simulink model "PMSM_Simscape_Model"  (R2020b)
settings: configuration reference "SLRT" (kept outside this file)
PreLoadFcn:
  | % Load modeSchedulerEnum if required
  | if ~exist('modeSchedulerEnum','class')
  |   load_system('ModeLogicModule');
  | end
undefined symbols (not defined in the file): adc, boardResistance, discInertia, encoder, inverter, pmsm, pmsmInertia, pwm
libraries: fl_lib x18, nesl_utility x10, ee_lib x3, eeTransforms x1
settings Model: DataDictionary=SGKitPlantData.sldd  EnableAccessToBaseWorkspace=off  OrderedModelArguments=off  Creator=promero  LastModifiedBy=manuel.fedou
settings ConfigSetRef: SourceName=SLRT

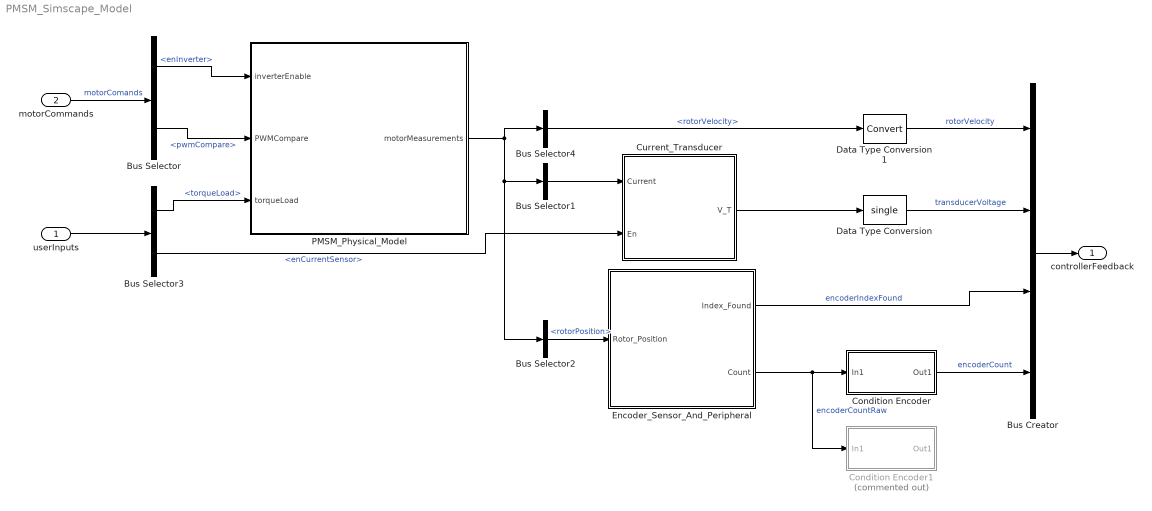
== system PMSM_Simscape_Model ==
  userInputs : Inport  OutDataTypeStr=Bus: userInputs  PortDimensions=1
  motorCommands : Inport  Port=2  OutDataTypeStr=Bus: motorCommands
  Bus Creator : BusCreator  Inputs=4  OutDataTypeStr=Bus: controllerFeedback
      settings: InheritFromInputs=off
  Bus Selector : BusSelector  OutputSignals=enInverter,pwmCompare
  Bus Selector1 : BusSelector  OutputSignals=phaseCurrentA,phaseCurrentB  OutputAsBus=on
  Bus Selector2 : BusSelector  OutputSignals=rotorPosition
  Bus Selector3 : BusSelector  OutputSignals=torqueLoad,enCurrentSensor
  Bus Selector4 : BusSelector  OutputSignals=rotorVelocity
  Condition Encoder : Subsystem  mask(Speedgoat Encoder Counter){cntsPerRevolution=encoder.CountPerRevolution, positiveDirection=encoder.ALeadsB}
      mask prompts: cntsPerRevolution "Counts per revolution"; positiveDirection "A leads B?"
      mask help: Configures the direction and positive range of the counter value returned by the Speedgoat IO313 QAD Read block.
      mask init:
      | if positiveDirection == 1
      |     strPositiveDirection = 'A Leads B';
      | else
      |     strPositiveDirection = 'B Leads A';
      | end
      mask Display: fprintf(['Encoder\nPositive Direction:\n' strPositiveDirection]);
  Condition Encoder1 : Subsystem  Commented=on  mask(Speedgoat Encoder Counter){cntsPerRevolution=encoder.CountPerRevolution, positiveDirection=encoder.ALeadsB}
      mask prompts: cntsPerRevolution "Counts per revolution"; positiveDirection "A leads B?"
      mask help: Configures the direction and positive range of the counter value returned by the Speedgoat IO313 QAD Read block.
      mask init:
      | if positiveDirection == 1
      |     strPositiveDirection = 'A Leads B';
      | else
      |     strPositiveDirection = 'B Leads A';
      | end
      mask Display: fprintf(['Encoder\nPositive Direction:\n' strPositiveDirection]);
  Current_Transducer : Subsystem
      mask Display: image('currentTransducerMask.png');
  Data Type Conversion : DataTypeConversion  OutDataTypeStr=single
  Data Type Conversion1 : DataTypeConversion
  Encoder_Sensor_And_Peripheral : Subsystem
      mask Display:
      | image('encoderSensorAndPeripheralMask.png')
      | port_label('input',1,'P')
      | port_label('output',1,sprintf('Index\nFound'))
      | port_label('output',2,'Count')
  PMSM_Physical_Model : Subsystem
      mask Display: image('focVelocityMotorAndLoadMask.png');
  controllerFeedback : Outport  OutDataTypeStr=Bus: controllerFeedback  VectorParamsAs1DForOutWhenUnconnected=off
  wires:
  Bus Selector3/1 -> PMSM_Physical_Model/3(torqueLoad)  "<torqueLoad>"
  Bus Selector2/1 -> Encoder_Sensor_And_Peripheral/1(Rotor_Position)  "<rotorPosition>"
  Bus Selector/2 -> PMSM_Physical_Model/2(PWMCompare)  "<pwmCompare>"
  motorCommands/1 -> Bus Selector/1  "motorComands"
  Encoder_Sensor_And_Peripheral/2(Count) -> Condition Encoder1/1(In1), Condition Encoder/1(In1)  "encoderCountRaw"
  Encoder_Sensor_And_Peripheral/1(Index_Found) -> Bus Creator/3  "encoderIndexFound"
  Bus Selector3/2 -> Current_Transducer/2(En)  "<enCurrentSensor>"
  Condition Encoder/1(Out1) -> Bus Creator/4  "encoderCount"
  Bus Selector1/1 -> Current_Transducer/1(Current)
  Bus Selector/1 -> PMSM_Physical_Model/1(inverterEnable)  "<enInverter>"
  userInputs/1 -> Bus Selector3/1
  Bus Creator/1 -> controllerFeedback/1
  PMSM_Physical_Model/1(motorMeasurements) -> Bus Selector4/1, Bus Selector2/1, Bus Selector1/1
  Current_Transducer/1(V_T) -> Data Type Conversion/1
  Data Type Conversion/1 -> Bus Creator/2  "transducerVoltage"
  Bus Selector4/1 -> Data Type Conversion1/1  "<rotorVelocity>"
  Data Type Conversion1/1 -> Bus Creator/1  "rotorVelocity"

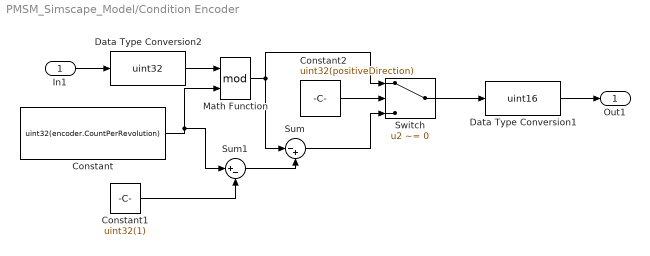
== system PMSM_Simscape_Model/Condition Encoder ==
  In1 : Inport
  Constant : Constant  Value=uint32(encoder.CountPerRevolution)  OutDataTypeStr=uint32
  Constant1 : Constant  Value=uint32(1)
  Constant2 : Constant  Value=uint32(positiveDirection)
  Data Type Conversion1 : DataTypeConversion  OutDataTypeStr=uint16
  Data Type Conversion2 : DataTypeConversion  OutDataTypeStr=uint32
  Math Function : Math  Operator=mod  SignedPower=on  SaturateOnIntegerOverflow=on
  Sum : Sum  Inputs=|-+
  Sum1 : Sum  Inputs=|+-
  Switch : Switch  Criteria=u2 ~= 0
  Out1 : Outport  VectorParamsAs1DForOutWhenUnconnected=off
  wires:
  Math Function/1 -> Sum/1, Switch/1
  Constant/1 -> Math Function/2, Sum1/1
  In1/1 -> Data Type Conversion2/1
  Data Type Conversion1/1 -> Out1/1
  Constant1/1 -> Sum1/2
  Sum1/1 -> Sum/2
  Constant2/1 -> Switch/2
  Sum/1 -> Switch/3
  Switch/1 -> Data Type Conversion1/1
  Data Type Conversion2/1 -> Math Function/1

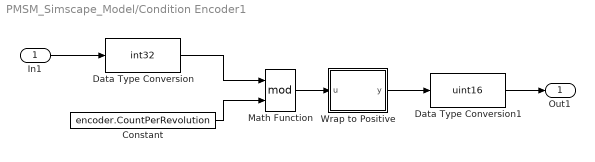
== system PMSM_Simscape_Model/Condition Encoder1 ==
  In1 : Inport
  Constant : Constant  Value=encoder.CountPerRevolution  OutDataTypeStr=int32
  Data Type Conversion : DataTypeConversion  OutDataTypeStr=int32
  Data Type Conversion1 : DataTypeConversion  OutDataTypeStr=uint16
  Math Function : Math  Operator=mod  SignedPower=on  SaturateOnIntegerOverflow=on
  Wrap to Positive : MATLAB Function  TreatAsAtomicUnit=on
  Out1 : Outport  VectorParamsAs1DForOutWhenUnconnected=off
  wires:
  Math Function/1 -> Wrap to Positive/1(u)
  Constant/1 -> Math Function/2
  In1/1 -> Data Type Conversion/1
  Wrap to Positive/1(y) -> Data Type Conversion1/1
  Data Type Conversion/1 -> Math Function/1
  Data Type Conversion1/1 -> Out1/1

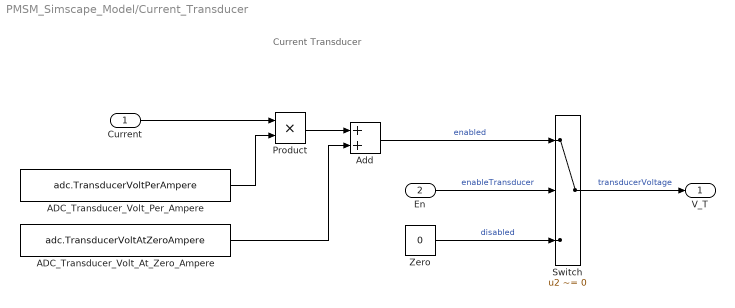
== system PMSM_Simscape_Model/Current_Transducer ==
  note: Current Transducer
  Current : Inport
  En : Inport  Port=2
  ADC_Transducer_Volt_At_Zero_Ampere : Constant  Value=adc.TransducerVoltAtZeroAmpere
  ADC_Transducer_Volt_Per_Ampere : Constant  Value=adc.TransducerVoltPerAmpere
  Add : Sum
  Product : Product  RndMeth=Zero
  Switch : Switch  Criteria=u2 ~= 0
  Zero : Constant  Value=0
  V_T : Outport  VectorParamsAs1DForOutWhenUnconnected=off
  wires:
  Current/1 -> Product/1
  ADC_Transducer_Volt_At_Zero_Ampere/1 -> Add/2
  Product/1 -> Add/1
  ADC_Transducer_Volt_Per_Ampere/1 -> Product/2
  Zero/1 -> Switch/3  "disabled"
  Switch/1 -> V_T/1  "transducerVoltage"
  Add/1 -> Switch/1  "enabled"
  En/1 -> Switch/2  "enableTransducer"

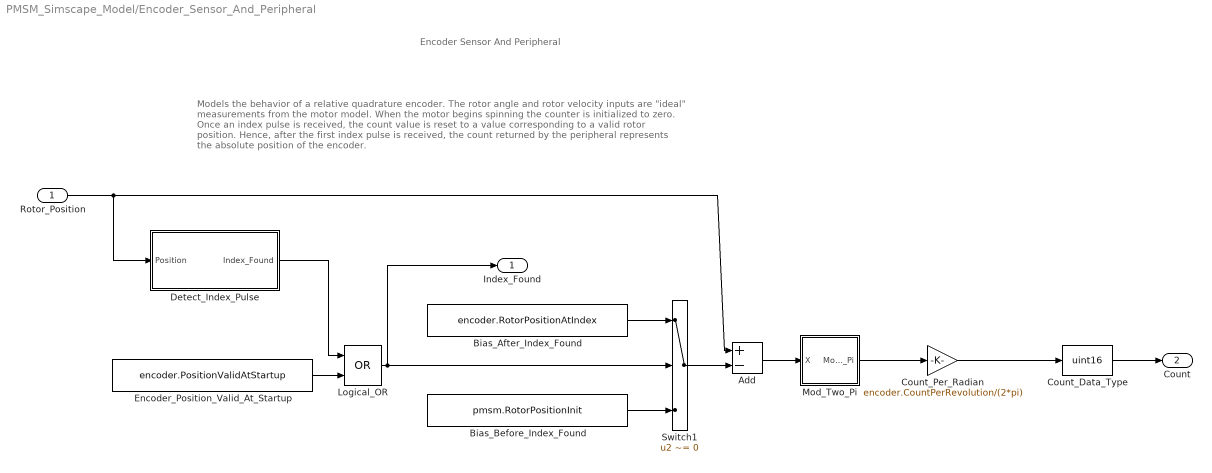
== system PMSM_Simscape_Model/Encoder_Sensor_And_Peripheral ==
  note: Models the behavior of a relative quadrature encoder. The rotor angle and rotor velocity inputs are "ideal" measurements from the motor model.
      | When the motor begins spinning the counter is initialized to zero.
      | Once an index pulse is received, the count value is reset to a value corresponding to a valid rotor position.
      | Hence, after the first index pulse is received, the count returned by the peripheral represents the absolute position of the encoder.
  note: Encoder Sensor And Peripheral
  Rotor_Position : Inport
  Add : Sum  Inputs=+-
  Bias_After_Index_Found : Constant  Value=encoder.RotorPositionAtIndex
  Bias_Before_Index_Found : Constant  Value=pmsm.RotorPositionInit
  Count_Data_Type : DataTypeConversion  OutDataTypeStr=uint16
  Count_Per_Radian : Gain  Gain=encoder.CountPerRevolution/(2*pi)
      settings: AttributesFormatString=|
      | ------------------------------------------
      | Gain = %<Gain>
  Detect_Index_Pulse : Subsystem
  Encoder_Position_Valid_At_Startup : Constant  Value=encoder.PositionValidAtStartup
  Logical_OR : Logic  Operator=OR  IconShape=distinctive  AllPortsSameDT=off  OutDataTypeStr=boolean
  Mod_Two_Pi : Subsystem
      mask Display:
      | text(0.5, 0.5,'Mod 2\pi',...
      |   'HorizontalAlignment', 'Center',...
      |   'VerticalAlignment', 'Middle',...
      |   'texmode', 'on')
  Switch1 : Switch  Criteria=u2 ~= 0
  Index_Found : Outport  VectorParamsAs1DForOutWhenUnconnected=off
  Count : Outport  Port=2  VectorParamsAs1DForOutWhenUnconnected=off
  wires:
  Bias_Before_Index_Found/1 -> Switch1/3
  Bias_After_Index_Found/1 -> Switch1/1
  Logical_OR/1 -> Index_Found/1, Switch1/2
  Encoder_Position_Valid_At_Startup/1 -> Logical_OR/2
  Detect_Index_Pulse/1(Index_Found) -> Logical_OR/1
  Rotor_Position/1 -> Add/1, Detect_Index_Pulse/1(Position)
  Mod_Two_Pi/1(Mod_X_Two_Pi) -> Count_Per_Radian/1
  Count_Data_Type/1 -> Count/1
  Switch1/1 -> Add/2
  Add/1 -> Mod_Two_Pi/1(X)
  Count_Per_Radian/1 -> Count_Data_Type/1

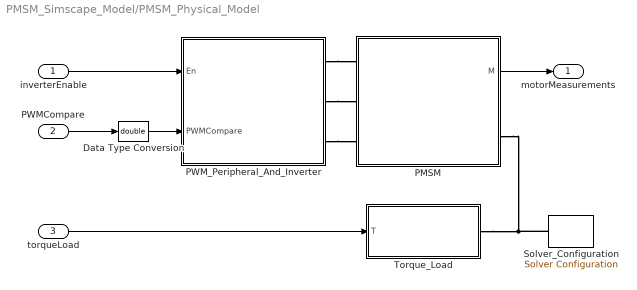
== system PMSM_Simscape_Model/PMSM_Physical_Model ==
  inverterEnable : Inport
  PWMCompare : Inport  Port=2
  torqueLoad : Inport  Port=3
  Data Type Conversion : DataTypeConversion  OutDataTypeStr=double
  PMSM : Subsystem
      mask Display:
      | image('pmsmMask.png')
      | text(0.03, 0.80, 'A', 'HorizontalAlignment', 'Left')
      | text(0.03, 0.50, 'B', 'HorizontalAlignment', 'Left')
      | text(0.03, 0.20, 'C', 'HorizontalAlignment', 'Left')
      | text(0.98, 0.75, 'M', 'HorizontalAlignment', 'Right')
      | text(0.98, 0.25, 'R', 'HorizontalAlignment', 'Right')
  PWM_Peripheral_And_Inverter : Subsystem  VariantControl=variantPwm == enumPwm.behavior
      mask Display: image('pwmPeripheralAndInverterMask.png');
  Solver_Configuration : nesl_utility/Solver Configuration  PhysicalDomain=network_engine_domain  SubClassName=solver  LeftPortType=input  RightPortType=generic  Tones=[]  Harmonics=[]  SimulateNoise=off  Profile=off  UseLocalSampling=off  EnableSwitchedLinearOptims=on  FrequencyDomain=off  UseCCode=off  RelTol=0.001  AbsTol=1e-06  MinStep=1e-09  ToWorkspace=off  RevertToSquareIcSolve=off  NumHomotopyIterations=100  PhasorMode=off  PhasorModeNumHarmonics=1  DoDC=off  ResidualTolerance=1e-9  UseLocalSolver=on  LocalSolverChoice=NE_BACKWARD_EULER_ADVANCER  LocalSolverSampleTime=sampleTime.CurrentControl  DoFixedCost=on  MaxNonlinIter=1  MaxModeIter=2  ComputeImpulses=off  ImpulseIterations=2  LinearAlgebra=auto  EquationFormulation=NE_TIME_EF  DelaysMemoryBudget=1024  AutomaticFiltering=off  FilteringTimeConstant=0.001  PartitionStorageMethod=EXHAUSTIVE  PartitionMemoryBudget=1024  PartitionMethod=FAST
  Torque_Load : Subsystem  VariantControl=loadType == motorLoad.disc
      mask Display:
      | image('torqueLoadMask.png')
      | text(0.03, 0.5, 'T', 'HorizontalAlignment', 'Left')
      | text(0.98, 0.5, 'R', 'HorizontalAlignment', 'Right')
  motorMeasurements : Outport  VectorParamsAs1DForOutWhenUnconnected=off
  wires:
  PWMCompare/1 -> Data Type Conversion/1
  torqueLoad/1 -> Torque_Load/1(T)
  PMSM/1(M) -> motorMeasurements/1
  inverterEnable/1 -> PWM_Peripheral_And_Inverter/1(En)
  Data Type Conversion/1 -> PWM_Peripheral_And_Inverter/2(PWMCompare)
  connections:
  Solver_Configuration/RConn1 -- PMSM/RConn1 -- Torque_Load/RConn1
  PWM_Peripheral_And_Inverter/RConn3 -- PMSM/LConn3
  PWM_Peripheral_And_Inverter/RConn2 -- PMSM/LConn2
  PWM_Peripheral_And_Inverter/RConn1 -- PMSM/LConn1

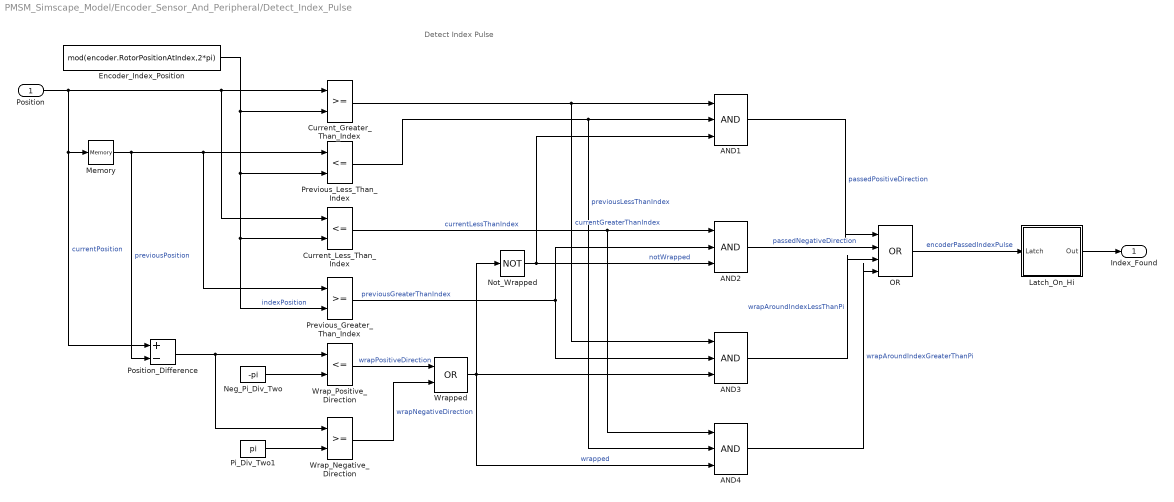
== system PMSM_Simscape_Model/Encoder_Sensor_And_Peripheral/Detect_Index_Pulse ==
  note: Detect Index Pulse
  Position : Inport
  AND{1..4} (4 alike) : Logic  Inputs=3  IconShape=distinctive  AllPortsSameDT=off  OutDataTypeStr=boolean
  Current_Greater_Than_Index : RelationalOperator  OutDataTypeStr=boolean  RndMeth=Nearest
  Current_Less_Than_Index : RelationalOperator  Operator=<=  OutDataTypeStr=boolean  RndMeth=Nearest
  Encoder_Index_Position : Constant  Value=mod(encoder.RotorPositionAtIndex,2*pi)
  Latch_On_Hi : Subsystem
  Memory : Memory  InheritSampleTime=on
  Neg_Pi_Div_Two : Constant  Value=-pi
  Not_Wrapped : Logic  Operator=NOT  IconShape=distinctive  AllPortsSameDT=off  OutDataTypeStr=boolean
  OR : Logic  Operator=OR  Inputs=4  IconShape=distinctive  AllPortsSameDT=off  OutDataTypeStr=boolean
  Pi_Div_Two1 : Constant  Value=pi
  Position_Difference : Sum  Inputs=+-
  Previous_Greater_Than_Index : RelationalOperator  OutDataTypeStr=boolean  RndMeth=Nearest
  Previous_Less_Than_Index : RelationalOperator  Operator=<=  OutDataTypeStr=boolean  RndMeth=Nearest
  Wrap_Negative_Direction : RelationalOperator  OutDataTypeStr=boolean  RndMeth=Nearest
  Wrap_Positive_Direction : RelationalOperator  Operator=<=  OutDataTypeStr=boolean  RndMeth=Nearest
  Wrapped : Logic  Operator=OR  IconShape=distinctive  AllPortsSameDT=off  OutDataTypeStr=boolean
  Index_Found : Outport  VectorParamsAs1DForOutWhenUnconnected=off
  wires:
  AND2/1 -> OR/2  "passedNegativeDirection"
  AND1/1 -> OR/1  "passedPositiveDirection"
  Current_Less_Than_Index/1 -> AND2/1, AND4/1  "currentLessThanIndex"
  Previous_Greater_Than_Index/1 -> AND2/2, AND3/2  "previousGreaterThanIndex"
  OR/1 -> Latch_On_Hi/1(Latch)  "encoderPassedIndexPulse"
  Encoder_Index_Position/1 -> Previous_Less_Than_Index/2, Previous_Greater_Than_Index/2, Current_Less_Than_Index/2, Current_Greater_Than_Index/2  "indexPosition"
  Previous_Less_Than_Index/1 -> AND1/2, AND4/2  "previousLessThanIndex"
  Current_Greater_Than_Index/1 -> AND3/1, AND1/1  "currentGreaterThanIndex"
  Memory/1 -> Position_Difference/2, Previous_Greater_Than_Index/1, Previous_Less_Than_Index/1  "previousPosition"
  Position/1 -> Memory/1, Position_Difference/1, Current_Less_Than_Index/1, Current_Greater_Than_Index/1  "currentPosition"
  Position_Difference/1 -> Wrap_Negative_Direction/1, Wrap_Positive_Direction/1
  Wrap_Positive_Direction/1 -> Wrapped/1  "wrapPositiveDirection"
  Neg_Pi_Div_Two/1 -> Wrap_Positive_Direction/2
  Wrap_Negative_Direction/1 -> Wrapped/2  "wrapNegativeDirection"
  Pi_Div_Two1/1 -> Wrap_Negative_Direction/2
  AND3/1 -> OR/3  "wrapAroundIndexLessThanPi"
  Latch_On_Hi/1(Out) -> Index_Found/1
  Not_Wrapped/1 -> AND1/3, AND2/3  "notWrapped"
  Wrapped/1 -> AND4/3, AND3/3, Not_Wrapped/1  "wrapped"
  AND4/1 -> OR/4  "wrapAroundIndexGreaterThanPi"

== system PMSM_Simscape_Model/Encoder_Sensor_And_Peripheral/Mod_Two_Pi ==
  note: Mod Two Pi
  X : Inport
  Mod : Math  Operator=mod  SignedPower=on  SaturateOnIntegerOverflow=on
  Two_Pi : Constant  Value=2*pi  OutDataTypeStr=Inherit: Inherit via back propagation
  Mod_X_Two_Pi : Outport  VectorParamsAs1DForOutWhenUnconnected=off
  wires:
  X/1 -> Mod/1
  Two_Pi/1 -> Mod/2
  Mod/1 -> Mod_X_Two_Pi/1

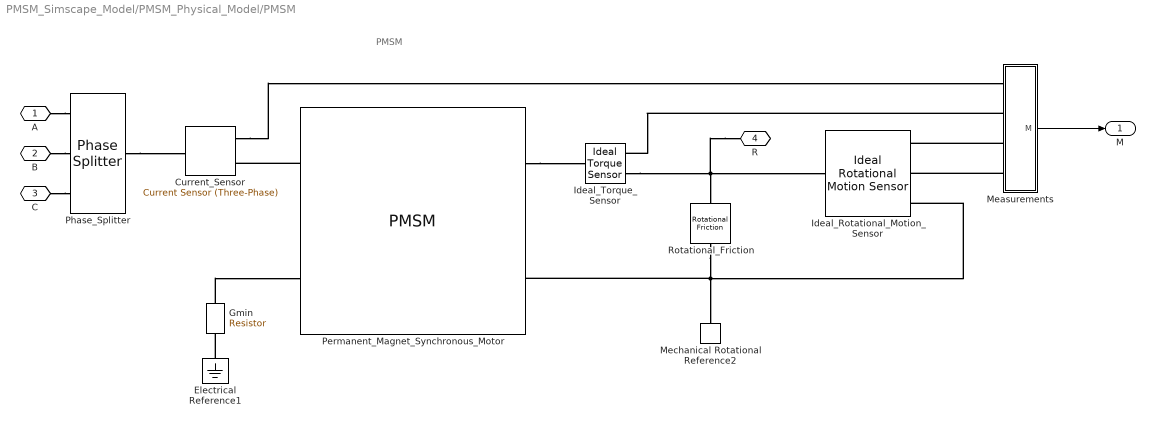
== system PMSM_Simscape_Model/PMSM_Physical_Model/PMSM ==
  note: PMSM
  Current_Sensor : ee_lib/Sensors & Transducers/Current Sensor (Three-Phase)
  Electrical Reference1 : fl_lib/Electrical/Electrical Elements/Electrical Reference
  Gmin : fl_lib/Electrical/Electrical Elements/Resistor  R=1e9 Ohm  i_specify=off  i_priority=None  i=0 A  i_nominal_specify=off  i_nominal_unit=A  i_nominal_value=1  v_specify=off  v_priority=None  v=0 V  v_nominal_specify=off  v_nominal_unit=V  v_nominal_value=1
  Ideal_Rotational_Motion_Sensor : fl_lib/Mechanical/Mechanical Sensors/Ideal Rotational Motion Sensor  wrap_angle=simscape.enum.onoff.off  offset=pmsm.RotorPositionInit rad
  Ideal_Torque_Sensor : fl_lib/Mechanical/Mechanical Sensors/Ideal Torque Sensor
  Measurements : Subsystem
  Mechanical Rotational Reference2 : fl_lib/Mechanical/Rotational Elements/Mechanical Rotational Reference
  Permanent_Magnet_Synchronous_Motor : ee_lib/Electromechanical/Permanent Magnet/PMSM  winding_type=ee.enum.statorconnection.wye  machine_param=ee.enum.pmsm.parameterization.constant  nPolePairs=pmsm.PolePairs  pmflux_param=ee.enum.pmflux.fluxlinkage  pm_flux_linkage=pmsm.FluxLinkage Wb  torque_constant=pmsm.TorqueConstant N*m/A  back_emf_constant=0.18 V/(rad/s)  stator_param=ee.enum.statorparam.LdLqL0  Ld=pmsm.InductanceLd H  Lq=pmsm.InductanceLq H  idVec=[-200, 0, 200] A  iqVec=[-200, 0, 200] A  LdMatrix=0.0002 * ones(3, 3) H  LqMatrix=0.0002 * ones(3, 3) H  PmMatrix=0.1 * ones(3, 3) Wb  ktMatrix=0.18 * ones(3, 3) N*m/A  keMatrix=0.18 * ones(3, 3) V/(rad/s)  L0=pmsm.InductanceL0 H  Ls=0.0002 H  Lm=0 H  Ms=0 H  Rs=pmsm.StatorPhaseResistance Ohm  zero_sequence=ee.enum.park.zerosequence.exclude  J=pmsmInertia+discInertia kg*m^2  lam=0 N*m/(rad/s)  axes_param=ee.enum.rotorangle.daxis  i_d_specify=off  i_d_priority=None  i_d=0 A  i_d_nominal_specify=off  i_d_nominal_unit=A  i_d_nominal_value=1  i_q_specify=off  i_q_priority=None  i_q=0 A  i_q_nominal_specify=off  i_q_nominal_unit=A  i_q_nominal_value=1  torque_specify=off  torque_priority=None  torque=0 N*m  torque_nominal_specify=off  torque_nominal_unit=N*m  torque_nominal_value=1  angular_velocity_specify=on  angular_velocity_priority=High  angular_velocity=pmsm.RotorVelocityInit rad/s  angular_velocity_nominal_specify=off  angular_velocity_nominal_unit=rpm  angular_velocity_nominal_value=1  angular_position_specify=on  angular_position_priority=High  angular_position=pmsm.RotorPositionInit rad  angular_position_nominal_specify=off  angular_position_nominal_unit=deg  angular_position_nominal_value=1  loss_param=ee.enum.ironloss.none  losses_oc=[0, 0, 0] W  losses_sc=[0, 0, 0] W  f_losses=60 Hz  Isc_losses=95 A  Tmeas=298.15 K  alpha=3.93e-3 1/K  alpha_flux=-0.001 1/K  stator_thermal_mass=100 J/K  rotor_thermal_mass=200 J/K  Rm_percent_rotor=90  Rd_percent_rotor=30  temperatureA_specify=off  temperatureA_priority=High  temperatureA=25 degC  temperatureA_nominal_specify=off  temperatureA_nominal_unit=degC  temperatureA_nominal_value=1  temperatureB_specify=off  temperatureB_priority=High  temperatureB=25 degC  temperatureB_nominal_specify=off  temperatureB_nominal_unit=degC  temperatureB_nominal_value=1  temperatureC_specify=off  temperatureC_priority=High  temperatureC=25 degC  temperatureC_nominal_specify=off  temperatureC_nominal_unit=degC  temperatureC_nominal_value=1  temperatureR_specify=off  temperatureR_priority=High  temperatureR=25 degC  temperatureR_nominal_specify=off  temperatureR_nominal_unit=degC  temperatureR_nominal_value=1
      settings: InternalSimscapePortConfiguration="{\"Bottom\":[],\"Left\":[{\"id\":\"N\",\"label\":\"~\",\"type\":\"foundation.electrical.three_phase\"},{\"id\":\"n\",\"label\":\"n\",\"type\":\"foundation.electrical.electrical\"}],\"Right\":[{\"id\":\"R\",\"label\":\"R\",\"type\":\"foundation.mechanical.rotational.rotational\"},{\"id\":\"C\",\"label\":\"C\",\"type\":\"foundation.mechanical.rotational.rotational\"}],\"Top\":[]}"
  Phase_Splitter : ee_lib/Connectors & References/Phase Splitter
      settings: SourceProductBaseCode=PS
  Rotational_Friction : fl_lib/Mechanical/Rotational Elements/Rotational Friction  brkwy_trq=pmsmBreakawayFrictionTorque N*m  brkwy_vel=pmsmBreakawayFrictionVelocity rad/s  Col_trq=pmsmCoulombFrictionTorque N*m  visc_coef=pmsmViscousFrictionCoefficient N*m/(rad/s)  w_specify=off  w_priority=None  w=0 rad/s  w_nominal_specify=off  w_nominal_unit=rad/s  w_nominal_value=1  t_specify=off  t_priority=None  t=0 N*m  t_nominal_specify=off  t_nominal_unit=N*m  t_nominal_value=1
  A : PMIOPort  Side=Left
  B : PMIOPort  Port=2  Side=Left
  C : PMIOPort  Port=3  Side=Left
  R : PMIOPort  Port=4  Side=Right
  M : Outport  VectorParamsAs1DForOutWhenUnconnected=off
  wires:
  Measurements/1(M) -> M/1
  connections:
  Measurements/LConn4 -- Ideal_Rotational_Motion_Sensor/RConn2
  Measurements/LConn3 -- Ideal_Rotational_Motion_Sensor/RConn3
  Measurements/LConn2 -- Ideal_Torque_Sensor/RConn2
  Permanent_Magnet_Synchronous_Motor/LConn1 -- Current_Sensor/RConn2
  C/RConn1 -- Phase_Splitter/RConn3
  B/RConn1 -- Phase_Splitter/RConn2
  A/RConn1 -- Phase_Splitter/RConn1
  Gmin/RConn1 -- Permanent_Magnet_Synchronous_Motor/LConn2
  Permanent_Magnet_Synchronous_Motor/RConn2 -- Rotational_Friction/RConn1 -- Ideal_Rotational_Motion_Sensor/RConn1 -- Mechanical Rotational Reference2/LConn1
  Phase_Splitter/LConn1 -- Current_Sensor/LConn1
  Current_Sensor/RConn1 -- Measurements/LConn1
  Electrical Reference1/LConn1 -- Gmin/LConn1
  Permanent_Magnet_Synchronous_Motor/RConn1 -- Ideal_Torque_Sensor/LConn1
  R/RConn1 -- Ideal_Rotational_Motion_Sensor/LConn1 -- Ideal_Torque_Sensor/RConn1 -- Rotational_Friction/LConn1

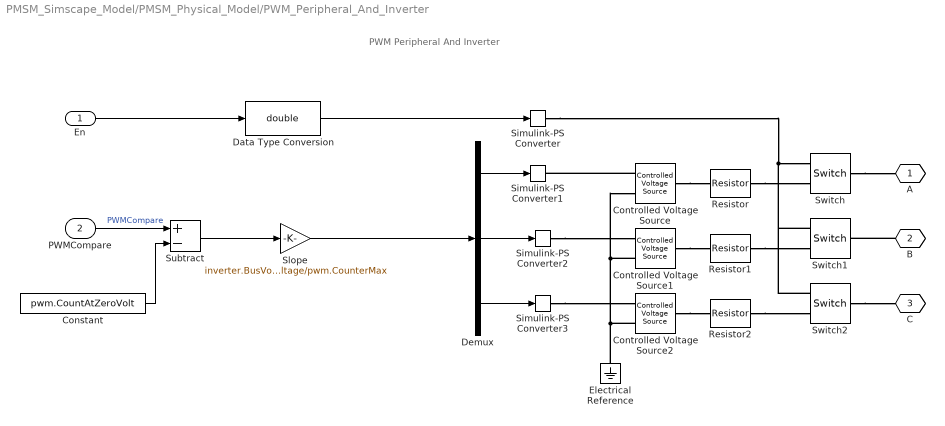
== system PMSM_Simscape_Model/PMSM_Physical_Model/PWM_Peripheral_And_Inverter ==
  note: PWM Peripheral And Inverter
  En : Inport
  PWMCompare : Inport  Port=2
  Constant : Constant  Value=pwm.CountAtZeroVolt  SampleTime=-1
  Controlled Voltage Source : fl_lib/Electrical/Electrical Sources/Controlled Voltage Source
  Controlled Voltage Source1 : fl_lib/Electrical/Electrical Sources/Controlled Voltage Source
  Controlled Voltage Source2 : fl_lib/Electrical/Electrical Sources/Controlled Voltage Source
  Data Type Conversion : DataTypeConversion  OutDataTypeStr=double
  Demux : Demux  Outputs=3
  Electrical Reference : fl_lib/Electrical/Electrical Elements/Electrical Reference
  Resistor : fl_lib/Electrical/Electrical Elements/Resistor  R=boardResistance Ohm  i_specify=off  i_priority=None  i=0 A  i_nominal_specify=off  i_nominal_unit=A  i_nominal_value=1  v_specify=off  v_priority=None  v=0 V  v_nominal_specify=off  v_nominal_unit=V  v_nominal_value=1
  Resistor1 : fl_lib/Electrical/Electrical Elements/Resistor  R=boardResistance Ohm  i_specify=off  i_priority=None  i=0 A  i_nominal_specify=off  i_nominal_unit=A  i_nominal_value=1  v_specify=off  v_priority=None  v=0 V  v_nominal_specify=off  v_nominal_unit=V  v_nominal_value=1
  Resistor2 : fl_lib/Electrical/Electrical Elements/Resistor  R=boardResistance Ohm  i_specify=off  i_priority=None  i=0 A  i_nominal_specify=off  i_nominal_unit=A  i_nominal_value=1  v_specify=off  v_priority=None  v=0 V  v_nominal_specify=off  v_nominal_unit=V  v_nominal_value=1
  Simulink-PS Converter : nesl_utility/Simulink-PS Converter  PhysicalDomain=network_engine_domain  SubClassName=ps_input  LeftPortType=input  RightPortType=output  PseudoPeriodic=off  Frequencies=[]  NoiseDistribution=none  NoiseParameters=[]  Unit=1  AffineConversion=off  FilteringAndDerivatives=provide  SimscapeFilterOrder=1  InputFilterTimeConstant=0.001  UdotUserProvided=0
  Simulink-PS Converter1 : nesl_utility/Simulink-PS Converter  PhysicalDomain=network_engine_domain  SubClassName=ps_input  LeftPortType=input  RightPortType=output  PseudoPeriodic=off  Frequencies=[]  NoiseDistribution=none  NoiseParameters=[]  Unit=V  AffineConversion=off  FilteringAndDerivatives=provide  SimscapeFilterOrder=1  InputFilterTimeConstant=0.001  UdotUserProvided=0
  Simulink-PS Converter2 : nesl_utility/Simulink-PS Converter  PhysicalDomain=network_engine_domain  SubClassName=ps_input  LeftPortType=input  RightPortType=output  PseudoPeriodic=off  Frequencies=[]  NoiseDistribution=none  NoiseParameters=[]  Unit=V  AffineConversion=off  FilteringAndDerivatives=provide  SimscapeFilterOrder=1  InputFilterTimeConstant=0.001  UdotUserProvided=0
  Simulink-PS Converter3 : nesl_utility/Simulink-PS Converter  PhysicalDomain=network_engine_domain  SubClassName=ps_input  LeftPortType=input  RightPortType=output  PseudoPeriodic=off  Frequencies=[]  NoiseDistribution=none  NoiseParameters=[]  Unit=V  AffineConversion=off  FilteringAndDerivatives=provide  SimscapeFilterOrder=1  InputFilterTimeConstant=0.001  UdotUserProvided=0
  Slope : Gain  Gain=inverter.BusVoltage/pwm.CounterMax
      settings: AttributesFormatString=|
      | ----------------------------------------
      | Gain = %<Gain>
  Subtract : Sum  Inputs=+-
  Switch : fl_lib/Electrical/Electrical Elements/Switch  R_closed=0.01 Ohm  G_open=1e-8 1/Ohm  Threshold=0.5  i_specify=off  i_priority=None  i=0 A  i_nominal_specify=off  i_nominal_unit=A  i_nominal_value=1  v_specify=off  v_priority=None  v=0 V  v_nominal_specify=off  v_nominal_unit=V  v_nominal_value=1
  Switch1 : fl_lib/Electrical/Electrical Elements/Switch  R_closed=0.01 Ohm  G_open=1e-8 1/Ohm  Threshold=0.5  i_specify=off  i_priority=None  i=0 A  i_nominal_specify=off  i_nominal_unit=A  i_nominal_value=1  v_specify=off  v_priority=None  v=0 V  v_nominal_specify=off  v_nominal_unit=V  v_nominal_value=1
  Switch2 : fl_lib/Electrical/Electrical Elements/Switch  R_closed=0.01 Ohm  G_open=1e-8 1/Ohm  Threshold=0.5  i_specify=off  i_priority=None  i=0 A  i_nominal_specify=off  i_nominal_unit=A  i_nominal_value=1  v_specify=off  v_priority=None  v=0 V  v_nominal_specify=off  v_nominal_unit=V  v_nominal_value=1
  A : PMIOPort  Tag=PMCPort  Side=Right
  B : PMIOPort  Tag=PMCPort  Port=2  Side=Right
  C : PMIOPort  Tag=PMCPort  Port=3  Side=Right
  wires:
  En/1 -> Data Type Conversion/1
  Slope/1 -> Demux/1
  PWMCompare/1 -> Subtract/1  "PWMCompare"
  Demux/1 -> Simulink-PS Converter1/1
  Demux/2 -> Simulink-PS Converter2/1
  Demux/3 -> Simulink-PS Converter3/1
  Data Type Conversion/1 -> Simulink-PS Converter/1
  Subtract/1 -> Slope/1
  Constant/1 -> Subtract/2
  connections:
  Controlled Voltage Source2/LConn1 -- Resistor2/LConn1
  Resistor1/RConn1 -- Switch1/RConn2
  Resistor/RConn1 -- Switch/RConn2
  Electrical Reference/LConn1 -- Controlled Voltage Source1/RConn2 -- Controlled Voltage Source/RConn2 -- Controlled Voltage Source2/RConn2
  Switch/LConn1 -- A/RConn1
  B/RConn1 -- Switch1/LConn1
  Simulink-PS Converter/RConn1 -- Switch2/RConn1 -- Switch1/RConn1 -- Switch/RConn1
  Switch2/LConn1 -- C/RConn1
  Controlled Voltage Source/RConn1 -- Simulink-PS Converter1/RConn1
  Simulink-PS Converter2/RConn1 -- Controlled Voltage Source1/RConn1
  Simulink-PS Converter3/RConn1 -- Controlled Voltage Source2/RConn1
  Controlled Voltage Source/LConn1 -- Resistor/LConn1
  Controlled Voltage Source1/LConn1 -- Resistor1/LConn1
  Resistor2/RConn1 -- Switch2/RConn2

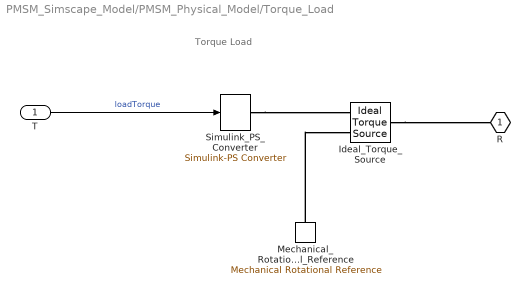
== system PMSM_Simscape_Model/PMSM_Physical_Model/Torque_Load ==
  note: Torque Load
  T : Inport
  Ideal_Torque_Source : fl_lib/Mechanical/Mechanical Sources/Ideal Torque Source
  Mechanical_Rotational_Reference : fl_lib/Mechanical/Rotational Elements/Mechanical Rotational Reference
  Simulink_PS_Converter : nesl_utility/Simulink-PS Converter  PhysicalDomain=network_engine_domain  SubClassName=ps_input  LeftPortType=input  RightPortType=output  PseudoPeriodic=off  Frequencies=[]  NoiseDistribution=none  NoiseParameters=[]  Unit=N*m  AffineConversion=off  FilteringAndDerivatives=zero  SimscapeFilterOrder=1  InputFilterTimeConstant=.001  UdotUserProvided=0
  R : PMIOPort  Side=Right
  wires:
  T/1 -> Simulink_PS_Converter/1  "loadTorque"
  connections:
  Ideal_Torque_Source/LConn1 -- R/RConn1
  Simulink_PS_Converter/RConn1 -- Ideal_Torque_Source/RConn1
  Mechanical_Rotational_Reference/LConn1 -- Ideal_Torque_Source/RConn2

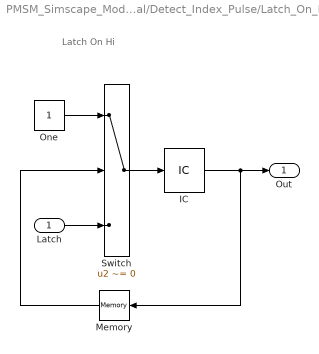
== system PMSM_Simscape_Model/Encoder_Sensor_And_Peripheral/Detect_Index_Pulse/Latch_On_Hi ==
  note: Latch On Hi
  Latch : Inport
  IC : InitialCondition  Value=0
  Memory : Memory  InheritSampleTime=on
  One : Constant  OutDataTypeStr=boolean
  Switch : Switch  Criteria=u2 ~= 0  Threshold=1
  Out : Outport  VectorParamsAs1DForOutWhenUnconnected=off
  wires:
  IC/1 -> Memory/1, Out/1
  Latch/1 -> Switch/3
  Switch/1 -> IC/1
  One/1 -> Switch/1
  Memory/1 -> Switch/2

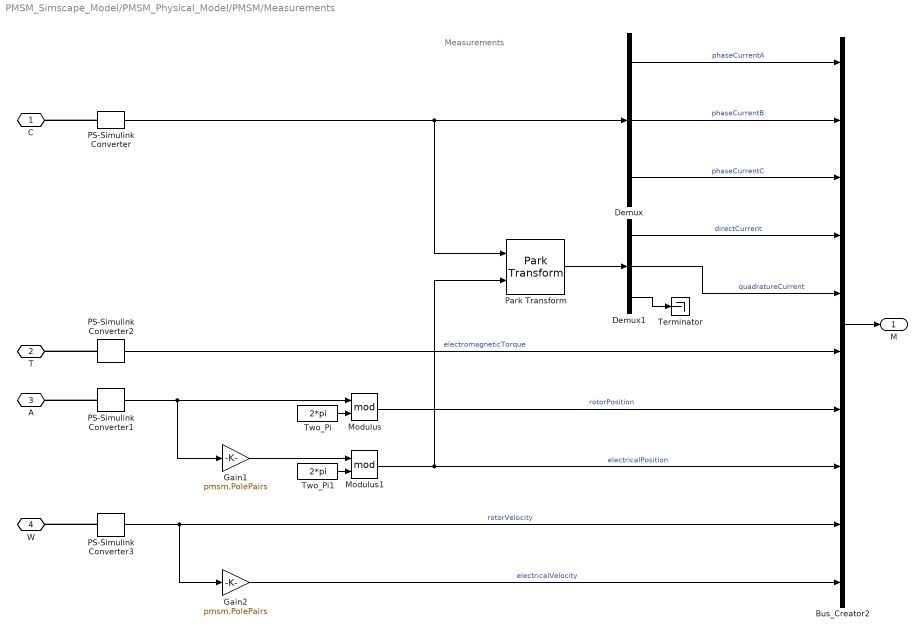
== system PMSM_Simscape_Model/PMSM_Physical_Model/PMSM/Measurements ==
  note: Measurements
  Bus_Creator2 : BusCreator  Inputs=10
  Demux : Demux  Outputs=3
  Demux1 : Demux  Outputs=3
  Gain1 : Gain  Gain=pmsm.PolePairs
      settings: AttributesFormatString=-----------------------------\n%<Gain>
  Gain2 : Gain  Gain=pmsm.PolePairs
      settings: AttributesFormatString=-----------------------------\n%<Gain>
  Modulus : Math  Operator=mod  SignedPower=on  SaturateOnIntegerOverflow=on
  Modulus1 : Math  Operator=mod  SignedPower=on  SaturateOnIntegerOverflow=on
  PS-Simulink Converter : nesl_utility/PS-Simulink Converter  PhysicalDomain=network_engine_domain  SubClassName=ps_output  LeftPortType=input  RightPortType=output  PseudoPeriodic=off  Frequencies=[]  Unit=A  AffineConversion=off
  PS-Simulink Converter1 : nesl_utility/PS-Simulink Converter  PhysicalDomain=network_engine_domain  SubClassName=ps_output  LeftPortType=input  RightPortType=output  PseudoPeriodic=off  Frequencies=[]  Unit=rad  AffineConversion=off
  PS-Simulink Converter2 : nesl_utility/PS-Simulink Converter  PhysicalDomain=network_engine_domain  SubClassName=ps_output  LeftPortType=input  RightPortType=output  PseudoPeriodic=off  Frequencies=[]  Unit=N*m  AffineConversion=off
  PS-Simulink Converter3 : nesl_utility/PS-Simulink Converter  PhysicalDomain=network_engine_domain  SubClassName=ps_output  LeftPortType=input  RightPortType=output  PseudoPeriodic=off  Frequencies=[]  Unit=rad/s  AffineConversion=off
  Park Transform : eeTransforms/Park Transform  AxisAlignment=D-axis  PowerInvariant=off
  Terminator : Terminator
  Two_Pi : Constant  Value=2*pi  OutDataTypeStr=Inherit: Inherit via back propagation
  Two_Pi1 : Constant  Value=2*pi  OutDataTypeStr=Inherit: Inherit via back propagation
  C : PMIOPort  Side=Left
  T : PMIOPort  Port=2  Side=Left
  A : PMIOPort  Port=3  Side=Left
  W : PMIOPort  Port=4  Side=Left
  M : Outport  OutDataTypeStr=Bus: motorMeasurements  VectorParamsAs1DForOutWhenUnconnected=off
  wires:
  Demux/2 -> Bus_Creator2/2  "phaseCurrentB"
  Demux/3 -> Bus_Creator2/3  "phaseCurrentC"
  Demux/1 -> Bus_Creator2/1  "phaseCurrentA"
  PS-Simulink Converter/1 -> Park Transform/1, Demux/1
  Bus_Creator2/1 -> M/1
  PS-Simulink Converter2/1 -> Bus_Creator2/6  "electromagneticTorque"
  PS-Simulink Converter3/1 -> Bus_Creator2/9, Gain2/1  "rotorVelocity"
  Modulus/1 -> Bus_Creator2/7  "rotorPosition"
  Modulus1/1 -> Park Transform/2, Bus_Creator2/8  "electricalPosition"
  Gain2/1 -> Bus_Creator2/10  "electricalVelocity"
  Two_Pi/1 -> Modulus/2
  Two_Pi1/1 -> Modulus1/2
  Gain1/1 -> Modulus1/1
  PS-Simulink Converter1/1 -> Modulus/1, Gain1/1
  Demux1/1 -> Bus_Creator2/4  "directCurrent"
  Demux1/2 -> Bus_Creator2/5  "quadratureCurrent"
  Park Transform/1 -> Demux1/1
  Demux1/3 -> Terminator/1
  connections:
  PS-Simulink Converter/LConn1 -- C/RConn1
  PS-Simulink Converter1/LConn1 -- A/RConn1
  PS-Simulink Converter2/LConn1 -- T/RConn1
  PS-Simulink Converter3/LConn1 -- W/RConn1

== matlab function PMSM_Simscape_Model/Condition Encoder1/Wrap to Positive ==
  data: u input; y output; cntsPerRevolution parameter; positiveDirection parameter
function y = fcn(u,cntsPerRevolution,positiveDirection)
% Guarantee the count is between 0 and cntsPerRevolution
% (Speedgoat count can be negative)

% Simplest case
y=u;

% % Max consecutive index pulses that can be missed
% maxIndexPulseMissesToRecoverFrom = 2;
% 
% for index = 1:maxIndexPulseMissesToRecoverFrom
%     if y >= cntsPerRevolution
%         y = y - cntsPerRevolution;
%     elseif y < -cntsPerRevolution
%         y = y + cntsPerRevolution;
%     end
% end
% 
% % Wrap angle to positive value
% if (y<0)
%     y = cntsPerRevolution + y;
% end

% Handle case of swapping encoder A & B signals
if positiveDirection ~= 1
    y = (cntsPerRevolution-1) - y;
end
